simulink model "tev5sim"  (Simulink 3.00)
settings: Solver=ode1  SolverMode=SingleTasking  StartTime=0.0  StopTime=0.3  FixedStep=1/3600  RelTol=1e-3  AbsTol=1e-6
settings Model: LastModifiedBy=default

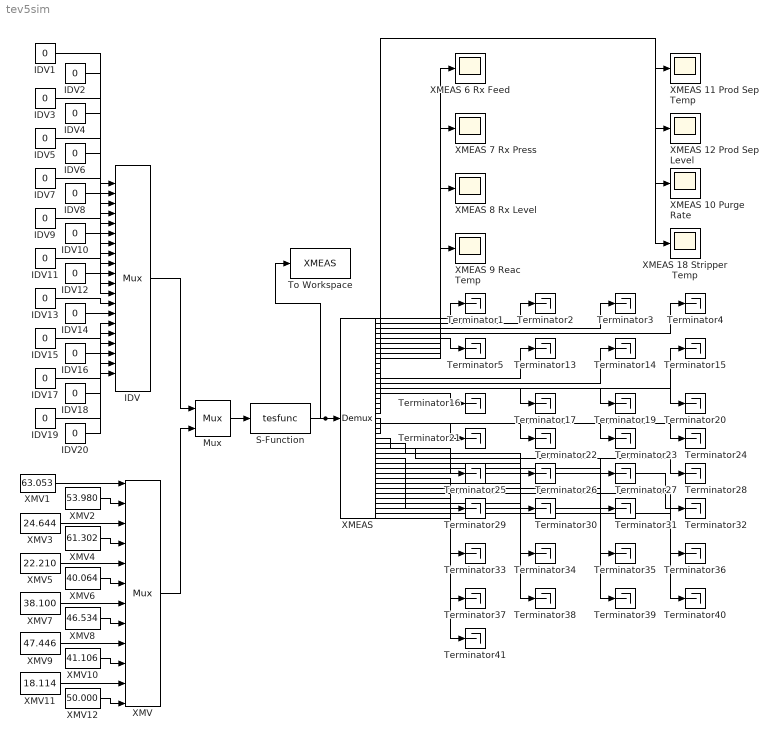
== system tev5sim ==
  IDV : Mux  Inputs=20
      settings: DisplayOption=none
  IDV{1..20} (20 alike) : Constant  Value=0
  Mux : Mux  Inputs=2
      settings: DisplayOption=none
  S-Function : S-Function  FunctionName=tesfunc  PortCounts=[]  SFunctionModules=''
  Terminator{1..5,13..17,19..41} (33 alike) : Terminator
  To Workspace : ToWorkspace  VariableName=XMEAS  SampleTime=-1  SaveFormat=Matrix
  XMEAS : Demux  Outputs=41
  XMEAS 10 Purge Rate : Scope
      settings: TickLabels=on  TimeRange=auto  YMin=0.29  YMax=0.35  SaveToWorkspace=off  SaveName=XMEAS10  DataFormat=Matrix
  XMEAS 11 Prod Sep Temp : Scope
      settings: TickLabels=on  TimeRange=auto  YMin=75  YMax=105  SaveToWorkspace=off  SaveName=XMEAS11  DataFormat=Matrix
  XMEAS 12 Prod Sep Level : Scope
      settings: TickLabels=on  TimeRange=auto  YMin=40  YMax=70  SaveToWorkspace=off  SaveName=XMEAS12  DataFormat=Matrix
  XMEAS 18 Stripper Temp : Scope
      settings: TickLabels=on  TimeRange=auto  YMin=65  YMax=74  SaveToWorkspace=off  SaveName=XMEAS18  DataFormat=Matrix
  XMEAS 6 Rx Feed : Scope
      settings: TickLabels=on  TimeRange=auto  YMin=39  YMax=43  SaveToWorkspace=off  SaveName=XMEAS6  DataFormat=Matrix
  XMEAS 7 Rx Press : Scope
      settings: TickLabels=on  TimeRange=auto  YMin=2500  YMax=2800  SaveToWorkspace=off  SaveName=XMEAS7  DataFormat=Matrix
  XMEAS 8 Rx Level : Scope
      settings: TickLabels=on  TimeRange=auto  YMin=72  YMax=77  SaveToWorkspace=off  SaveName=XMEAS8  DataFormat=Matrix
  XMEAS 9 Reac Temp : Scope
      settings: TickLabels=on  TimeRange=auto  YMin=120  YMax=140  SaveToWorkspace=off  SaveName=XMEAS9  DataFormat=Matrix
  XMV : Mux  Inputs=12
      settings: DisplayOption=none
  XMV1 : Constant  Value=63.053
  XMV10 : Constant  Value=41.106
  XMV11 : Constant  Value=18.114
  XMV12 : Constant  Value=50.000
  XMV2 : Constant  Value=53.980
  XMV3 : Constant  Value=24.644
  XMV4 : Constant  Value=61.302
  XMV5 : Constant  Value=22.210
  XMV6 : Constant  Value=40.064
  XMV7 : Constant  Value=38.100
  XMV8 : Constant  Value=46.534
  XMV9 : Constant  Value=47.446
  wires:
  IDV1/1 -> IDV/1
  IDV2/1 -> IDV/2
  IDV3/1 -> IDV/3
  IDV4/1 -> IDV/4
  IDV5/1 -> IDV/5
  IDV6/1 -> IDV/6
  IDV7/1 -> IDV/7
  IDV8/1 -> IDV/8
  IDV9/1 -> IDV/9
  IDV10/1 -> IDV/10
  IDV11/1 -> IDV/11
  IDV12/1 -> IDV/12
  IDV13/1 -> IDV/13
  IDV14/1 -> IDV/14
  IDV15/1 -> IDV/15
  IDV16/1 -> IDV/16
  IDV17/1 -> IDV/17
  IDV18/1 -> IDV/18
  IDV19/1 -> IDV/19
  IDV20/1 -> IDV/20
  XMV1/1 -> XMV/1
  XMV2/1 -> XMV/2
  XMV3/1 -> XMV/3
  XMV4/1 -> XMV/4
  XMV5/1 -> XMV/5
  XMV6/1 -> XMV/6
  XMV7/1 -> XMV/7
  XMV8/1 -> XMV/8
  XMV9/1 -> XMV/9
  XMV10/1 -> XMV/10
  XMV11/1 -> XMV/11
  XMV12/1 -> XMV/12
  IDV/1 -> Mux/1
  XMV/1 -> Mux/2
  Mux/1 -> S-Function/1
  XMEAS/1 -> Terminator1/1
  XMEAS/2 -> Terminator2/1
  XMEAS/3 -> Terminator3/1
  XMEAS/4 -> Terminator4/1
  XMEAS/5 -> Terminator5/1
  XMEAS/6 -> XMEAS 6 Rx Feed/1
  XMEAS/7 -> XMEAS 7 Rx Press/1
  XMEAS/8 -> XMEAS 8 Rx Level/1
  XMEAS/9 -> XMEAS 9 Reac Temp/1
  XMEAS/10 -> XMEAS 10 Purge Rate/1
  XMEAS/11 -> XMEAS 11 Prod Sep Temp/1
  XMEAS/12 -> XMEAS 12 Prod Sep Level/1
  XMEAS/13 -> Terminator13/1
  XMEAS/14 -> Terminator14/1
  XMEAS/15 -> Terminator15/1
  XMEAS/16 -> Terminator16/1
  XMEAS/17 -> Terminator17/1
  XMEAS/18 -> XMEAS 18 Stripper Temp/1
  XMEAS/19 -> Terminator19/1
  XMEAS/20 -> Terminator20/1
  XMEAS/21 -> Terminator21/1
  XMEAS/22 -> Terminator22/1
  XMEAS/23 -> Terminator23/1
  XMEAS/24 -> Terminator24/1
  XMEAS/25 -> Terminator25/1
  XMEAS/26 -> Terminator26/1
  XMEAS/27 -> Terminator27/1
  XMEAS/28 -> Terminator28/1
  XMEAS/29 -> Terminator29/1
  XMEAS/30 -> Terminator30/1
  XMEAS/31 -> Terminator31/1
  XMEAS/32 -> Terminator32/1
  XMEAS/33 -> Terminator33/1
  XMEAS/34 -> Terminator34/1
  XMEAS/35 -> Terminator35/1
  XMEAS/36 -> Terminator36/1
  XMEAS/37 -> Terminator37/1
  XMEAS/38 -> Terminator38/1
  XMEAS/39 -> Terminator39/1
  XMEAS/40 -> Terminator40/1
  XMEAS/41 -> Terminator41/1
  S-Function/1 -> XMEAS/1, To Workspace/1
